simulink model "edge_call_outputEvent_mulBrodcast_eg"  (R2020a)
settings: Solver=FixedStepAuto  StartTime=0.0  StopTime=10.0  FixedStep=1  MaxStep=1  RelTol=1e-3
settings Model: Creator=86188  LastModifiedBy=bzhan
settings DataIOCC: ReturnWorkspaceOutputs=off
settings DebuggingCC: ArithmeticOperatorsInVariantConditions=warning
settings SFSimCC: SimUseLocalCustomCode=off  CustomCodeUndefinedFunction=UseInterfaceOnly
settings RTWCC: RTWUseLocalCustomCode=off

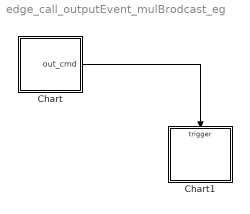
== system edge_call_outputEvent_mulBrodcast_eg ==
  Chart : Stateflow chart  TreatAsAtomicUnit=on
  Chart1 : Stateflow chart  TreatAsAtomicUnit=on
  wires:
  Chart/1(out_cmd) -> Chart1/Trigger

== stateflow chart edge_call_outputEvent_mulBrodcast_eg/Chart1 ==
  state AA
    en:f("en_AA");
    du:f("du_AA");
  (default) -> AA : {y = y + 1;}
  data: s function_input; y local =0
  events: out_cmd input EITHER_EDGE_EVENT
  function f(s):
    | function f(s)
    |   fprintf(s+"\n");

== stateflow chart edge_call_outputEvent_mulBrodcast_eg/Chart ==
  state ENTRY
    en:f("en_ENTRY");
  state A
    en:
    f("en_A");
    send(out_cmd);
    send(out_cmd);
    send(out_cmd);
    send(out_cmd);
  state B
  (default) -> ENTRY
  A -> B
  ENTRY -> A
  data: s function_input
  events: out_cmd output EITHER_EDGE_EVENT
  function f(s):
    | function f(s)
    |   fprintf(s+"\n");
